simulink subsystem "FilterOutFreq"  (R2023b)
settings: Solver=VariableStepAuto  StartTime=0.0  StopTime=10.0  RelTol=1e-3
settings Model: Creator=dfurodet  LastModifiedBy=dfurodet

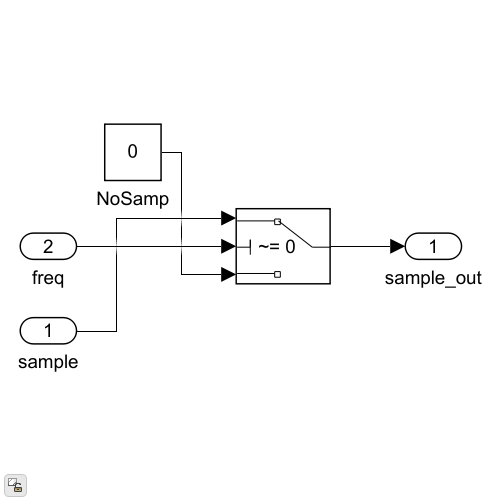
[thumbnail: Simulink's stored preview of the top-level diagram]
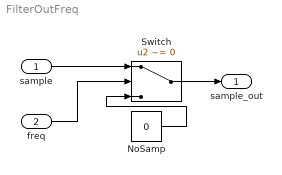
== system FilterOutFreq ==
  sample : Inport
  freq : Inport  Port=2
  NoSamp : Constant  Value=0
  Switch : Switch  Criteria=u2 ~= 0  SaturateOnIntegerOverflow=off  InputSameDT=off
  sample_out : Outport
  wires:
  freq/1 -> Switch/2
  NoSamp/1 -> Switch/3
  Switch/1 -> sample_out/1
  sample/1 -> Switch/1
